simulink model "frequencycountNewMethode"  (R2020a)
settings: Solver=ode45  StartTime=0.0  StopTime=50  FixedStep=5e-6  RelTol=1e-4  EnableMultiTasking=on
libraries: simulink x1
settings Model: ExtModeAutoUpdateStatusClock=off  Creator=mf  LastModifiedBy=Lukas Bilal
settings DataIOCC: LimitDataPoints=on  SaveFormat=Array  SignalLoggingSaveFormat=ModelDataLogs  ReturnWorkspaceOutputs=off  SignalLoggingName=sigsOut
settings OptimizationCC: BooleanDataType=off  ExpressionDepthLimit=2147483647  LifeSpan=inf
settings DebuggingCC: SaveWithParameterizedLinksMsg=none  UnderspecifiedInitializationDetection=Classic  MergeDetectMultiDrivingBlocksExec=none  SignalResolutionControl=TryResolveAllWithWarning  MultiTaskDSMMsg=warning  MultiTaskCondExecSysMsg=none  StateNameClashWarn=warning  SFUnexpectedBacktrackingDiag=warning  SFNoUnconditionalDefaultTransitionDiag=warning  SFExecutionAtInitializationDiag=none  ArithmeticOperatorsInVariantConditions=warning
settings HardwareCC: ProdBitPerPointer=32  ProdBitPerSizeT=32  ProdBitPerPtrDiffT=32  ProdLargestAtomicFloat=None  ProdIntDivRoundTo=Undefined  ProdEndianess=Unspecified  ProdWordSize=32  ProdHWDeviceType=32-bit Generic  TargetUnknown=on
settings ModelReferenceCC: PropagateSignalLabelsOutOfModel=off
settings SFSimCC: SimUseLocalCustomCode=off  SimParseCustomCode=off  CustomCodeUndefinedFunction=UseInterfaceOnly
settings RTWCC: RTWUseLocalCustomCode=off
settings CodeAppCC: StateflowObjectComments=on
settings GRTTargetCC: TargetLangStandard=C89/C90 (ANSI)  CombineOutputUpdateFcns=off  GRTInterface=on
settings ConfigComp: CovMetricSettings=dw  CovHtmlReporting=on  CovSaveCumulativeToWorkspaceVar=on  CovSaveSingleToWorkspaceVar=on  CovExternalEMLEnable=off

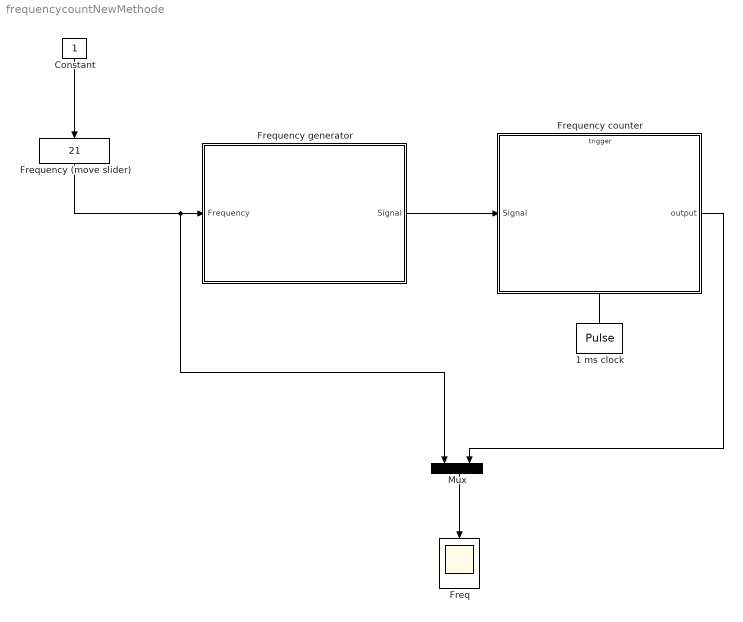
== system frequencycountNewMethode ==
  1 ms clock : DiscretePulseGenerator  PulseType=Time based  Period=1e-3  PulseWidth=50
  Constant : Constant
  Freq : Scope
  Frequency (move slider) : simulink/Math Operations/Slider Gain  gain=21  low=1  high=500
  Frequency counter : Stateflow chart  TreatAsAtomicUnit=on
  Frequency generator : Subsystem
  Mux : Mux  Inputs=2
  wires:
  Constant/1 -> Frequency (move slider)/1
  1 ms clock/1 -> Frequency counter/Trigger
  Mux/1 -> Freq/1
  Frequency (move slider)/1 -> Frequency generator/1(Frequency), Mux/1
  Frequency generator/1(Signal) -> Frequency counter/1(Signal)
  Frequency counter/1(output) -> Mux/2

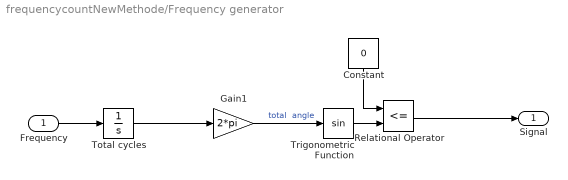
== system frequencycountNewMethode/Frequency generator ==
  Frequency : Inport
  Constant : Constant  Value=0
  Gain1 : Gain  Gain=2*pi  SaturateOnIntegerOverflow=on  OutDataTypeStr=Inherit: Same as input  ParamDataTypeStr=Inherit: Same as input
  Relational Operator : RelationalOperator  Operator=<=  OutDataTypeStr=boolean  RndMeth=Nearest
  Total cycles : Integrator
  Trigonometric Function : Trigonometry
  Signal : Outport
  wires:
  Frequency/1 -> Total cycles/1
  Trigonometric Function/1 -> Relational Operator/2
  Constant/1 -> Relational Operator/1
  Relational Operator/1 -> Signal/1
  Total cycles/1 -> Gain1/1
  Gain1/1 -> Trigonometric Function/1  "total  angle"

== stateflow chart frequencycountNewMethode/Frequency counter ==
  settings: executeAtInitialization=1
  state FrequencyCounter
    state FrequencyCounterMethode [parallel]
      settings: executionOrder=1
      state Clock [parallel]
        settings: executionOrder=2
        state Clock
        FrequencyCounter.FrequencyCounterMethode.Clock.Clock -> FrequencyCounter.FrequencyCounterMethode.Clock.Clock : clk [time < 1000]
            | {
            |   time++;
            | }  // Implementiert einfach
            |    // einen Timer.
      state Counter [parallel]
        settings: executionOrder=1
        state Counter
        FrequencyCounter.FrequencyCounterMethode.Counter.Counter -> FrequencyCounter.FrequencyCounterMethode.Counter.Counter [order 1] : [time == 1000]
            | {
            |   Measurement = counter;
            |   time = 0;
            |   counter = 0;
            |   flag++;
            | }
        FrequencyCounter.FrequencyCounterMethode.Counter.Counter -> FrequencyCounter.FrequencyCounterMethode.Counter.Counter [order 2] : [time < 1000 && Signal && hasChanged(Signal)]
            | {
            |   counter++;  // Zählt die Zyklen
            | }
    state FrequencyTimerMethode [parallel]
      settings: executionOrder=2
      state ClockStarter
      state FirstHigh
      state FirstLow
      (default) -> ClockStarter
      FirstHigh -> FirstLow [order 2] : [~Signal] / {cycles++;}
      FirstLow -> FirstLow [order 2] : [~Signal] / {cycles++;}
      ClockStarter -> FirstHigh : [Signal] /{cycles = 1;}
      FirstLow -> FirstHigh [order 1] : [Signal] {
          |   Measurement2 = 1000/cycles;  // 1000, weil die Periodendauer 1/10^-3 s = 1000 s
          |   cycles = 0;
          |   flag++;
          |  }
      FirstHigh -> FirstHigh [order 1] : [Signal] /{cycles++;}  // Solange kein low kam, vergehen Zyklen
    state Evaluation [parallel]
      settings: executionOrder=3
      state Test
      state Test2
      Test2 -> Test [order 2] : [Measurement >= 20] {
          |                                    output = Measurement;
          |                                    flag = 0;}
      (default) -> Test
      Test -> Test2 : [flag == 2]
      Test2 -> Test [order 1] : [Measurement < 20] {
          |                                    output = Measurement2;
          |                                    flag = 0;}
  (default) -> FrequencyCounter
  data: time local double =double(0); Signal input boolean; counter local double =double(0); cycles local double =double(0); output output double =0; flag local int8 =int8(0); Measurement local double =double(0); Measurement2 local double =double(0)
  events: clk input RISING_EDGE_EVENT
